simulink model "simpSubPlatform_th"  (R2018b)
settings: Solver=VariableStepAuto  StartTime=0.0  StopTime=sim_time  RelTol=1e-3
values from neighbouring files (symbols this model uses):
  Cd = 0.5    [simpSubPlatform_ts.m]
  dia_t = 0.05    [simpSubPlatform_ts.m]
  E = 3.8e9    (= 3800000000)    [simpSubPlatform_ts.m]
  flow = [.1 0 0]    [simpSubPlatform_ts.m]
  grav = 9.81    [simpSubPlatform_ts.m]
  initEulerAngles = [0 0 0]    [simpSubPlatform_ts.m]
  initPos = [0 0 100]    [simpSubPlatform_ts.m]
  mass = rho*vol/buoyF    (= 2692.30769231)    [simpSubPlatform_ts.m]
  rho = 1000    [simpSubPlatform_ts.m]
  rho_tether = 300    [simpSubPlatform_ts.m]
  tetherLengths = (norm(initPos+thr1Pt-thr1GndPos))*ones(3,1)    [simpSubPlatform_ts.m]
  thr1Pt = [0 1 -.5]    [simpSubPlatform_ts.m]
  thr2Pt = [cosd(30),-sind(30),-.5]    [simpSubPlatform_ts.m]
  thr3Pt = [-cosd(30),-sind(30),-.5]    [simpSubPlatform_ts.m]
  zeta = 0.05    [simpSubPlatform_ts.m]
undefined symbols (not defined in the file or in its folder): ini_Ri_o, ini_Vi_o, initNodePoss, initNodeVels, rotation_sequence, sim_param, singleTether_cl, Subsystem, Subsystem1, tetherBuoyancyAndWeight_ul, thr1Gnd, thr2Gnd, thr3Gnd, threeTethers_cl, zOcean
libraries: cylinderVolume_ul x3, tetherDragForce_ul x3, tetherInternalForces_ul x3, simpSubPlatform_cl x1, vectorNormalizer_ul x1
settings Model: Creator=Erin B  LastModifiedBy=Erin B

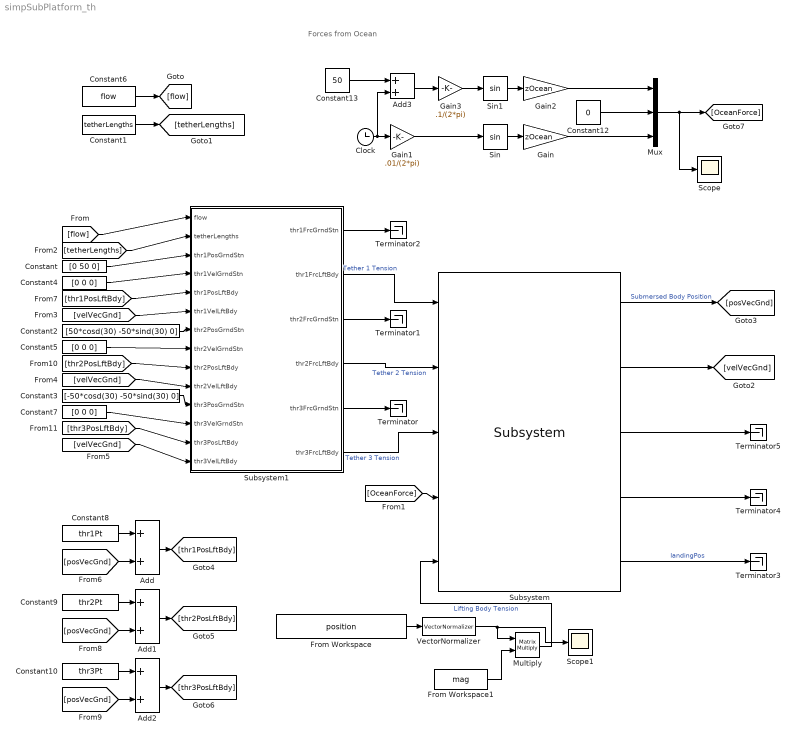
== system simpSubPlatform_th ==
  note: Forces from Ocean
  Add{,1..3} (4 alike) : Sum
  Clock : Clock
  Constant : Constant  Value=[0 50 0]
  Constant1 : Constant  Value=tetherLengths
  Constant10 : Constant  Value=thr3Pt
  Constant12 : Constant  Value=0
  Constant13 : Constant  Value=50
  Constant2 : Constant  Value=[50*cosd(30) -50*sind(30) 0]
  Constant3 : Constant  Value=[-50*cosd(30) -50*sind(30) 0]
  Constant4 : Constant  Value=[0 0 0]
  Constant5 : Constant  Value=[0 0 0]
  Constant6 : Constant  Value=flow
  Constant7 : Constant  Value=[0 0 0]
  Constant8 : Constant  Value=thr1Pt
  Constant9 : Constant  Value=thr2Pt
  From Workspace : FromWorkspace  VariableName=position  SampleTime=0
  From Workspace1 : FromWorkspace  VariableName=mag  SampleTime=0
  Gain : Gain  Gain=zOcean
  Gain1 : Gain  Gain=.01/(2*pi)
  Gain2 : Gain  Gain=zOcean
  Gain3 : Gain  Gain=.1/(2*pi)
  Multiply : Product  Multiplication=Matrix(*)
  Mux : Mux  Inputs=3
  Scope : Scope
  Scope1 : Scope
  Sin : Trigonometry  OutputSignalType=real
  Sin1 : Trigonometry  OutputSignalType=real
  Subsystem : simpSubPlatform_cl/Subsystem  SystemSampleTime=-1
  Subsystem1 : Subsystem  AncestorBlock=threeTethers_cl/Subsystem1
  Terminator{,1..5} (6 alike) : Terminator
  "VectorNormalizer " : vectorNormalizer_ul/VectorNormalizer   SystemSampleTime=-1
  wires:
  Subsystem1/4(thr2FrcLftBdy) -> Subsystem/2  "Tether 2 Tension"
  Subsystem1/5(thr3FrcGrndStn) -> Terminator/1
  Subsystem1/3(thr2FrcGrndStn) -> Terminator1/1
  Subsystem1/1(thr1FrcGrndStn) -> Terminator2/1
  Constant6/1 -> [flow]
  [flow] -> Subsystem1/1(flow)
  Constant1/1 -> [tetherLengths]
  [tetherLengths] -> Subsystem1/2(tetherLengths)
  Constant/1 -> Subsystem1/3(thr1PosGrndStn)
  Constant2/1 -> Subsystem1/7(thr2PosGrndStn)
  Constant3/1 -> Subsystem1/11(thr3PosGrndStn)
  Constant4/1 -> Subsystem1/4(thr1VelGrndStn)
  Constant5/1 -> Subsystem1/8(thr2VelGrndStn)
  Constant7/1 -> Subsystem1/12(thr3VelGrndStn)
  Subsystem/5 -> Terminator3/1  "landingPos"
  Subsystem/2 -> [velVecGnd]
  [velVecGnd] -> Subsystem1/6(thr1VelLftBdy)
  [velVecGnd] -> Subsystem1/10(thr2VelLftBdy)
  [velVecGnd] -> Subsystem1/14(thr3VelLftBdy)
  Constant8/1 -> Add/1
  Subsystem/1 -> [posVecGnd]  "Submersed Body Position"
  [posVecGnd] -> Add/2
  Add/1 -> [thr1PosLftBdy]
  [thr1PosLftBdy] -> Subsystem1/5(thr1PosLftBdy)
  Add1/1 -> [thr2PosLftBdy]
  Constant9/1 -> Add1/1
  [posVecGnd] -> Add1/2
  Add2/1 -> [thr3PosLftBdy]
  Constant10/1 -> Add2/1
  [posVecGnd] -> Add2/2
  [thr2PosLftBdy] -> Subsystem1/9(thr2PosLftBdy)
  [thr3PosLftBdy] -> Subsystem1/13(thr3PosLftBdy)
  Subsystem/4 -> Terminator4/1
  Subsystem/3 -> Terminator5/1
  Subsystem1/6(thr3FrcLftBdy) -> Subsystem/3  "Tether 3 Tension"
  Subsystem1/2(thr1FrcLftBdy) -> Subsystem/1  "Tether 1 Tension"
  Mux/1 -> Scope/1, [OceanForce]
  Sin/1 -> Gain/1
  Clock/1 -> Add3/2, Gain1/1
  [OceanForce] -> Subsystem/4
  Gain1/1 -> Sin/1
  Gain/1 -> Mux/3
  Constant13/1 -> Add3/1
  Add3/1 -> Gain3/1
  Sin1/1 -> Gain2/1
  Constant12/1 -> Mux/2
  Gain3/1 -> Sin1/1
  Gain2/1 -> Mux/1
  From Workspace/1 -> "VectorNormalizer "/1
  "VectorNormalizer "/1 -> Scope1/1, Multiply/1
  From Workspace1/1 -> Multiply/2
  Multiply/1 -> Subsystem/5  "Lifting Body Tension"

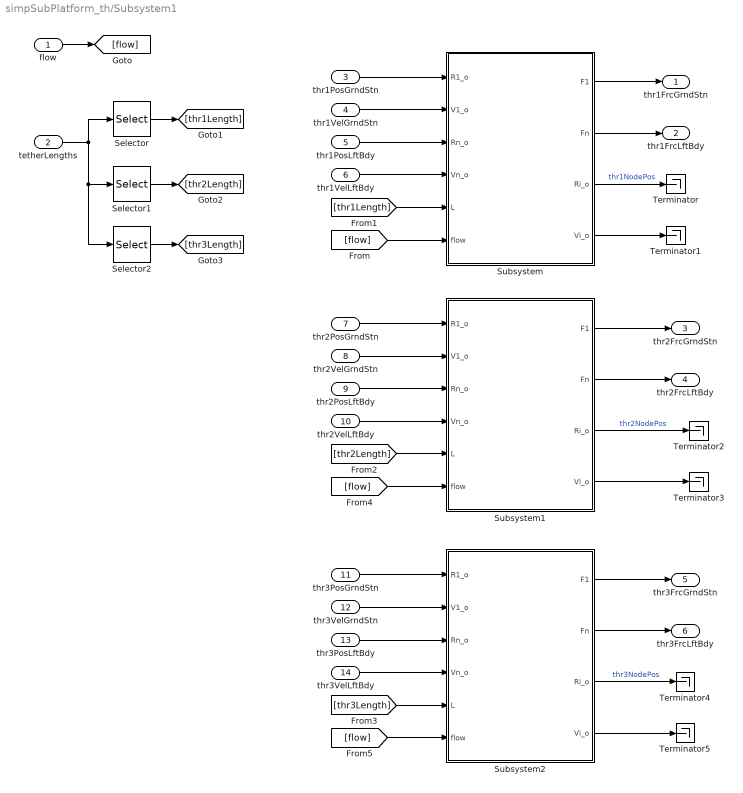
== system simpSubPlatform_th/Subsystem1 ==
  flow : Inport
  tetherLengths : Inport  Port=2
  thr1PosGrndStn : Inport  Port=3
  thr1VelGrndStn : Inport  Port=4
  thr1PosLftBdy : Inport  Port=5
  thr1VelLftBdy : Inport  Port=6
  thr2PosGrndStn : Inport  Port=7
  thr2VelGrndStn : Inport  Port=8
  thr2PosLftBdy : Inport  Port=9
  thr2VelLftBdy : Inport  Port=10
  thr3PosGrndStn : Inport  Port=11
  thr3VelGrndStn : Inport  Port=12
  thr3PosLftBdy : Inport  Port=13
  thr3VelLftBdy : Inport  Port=14
  Selector : Selector  InputPortWidth=3  IndexOptions=Index vector (dialog)  Indices=1  OutputSizes=1
  Selector1 : Selector  InputPortWidth=3  IndexOptions=Index vector (dialog)  Indices=2  OutputSizes=1
  Selector2 : Selector  InputPortWidth=3  IndexOptions=Index vector (dialog)  Indices=3  OutputSizes=1
  Subsystem : Subsystem  AncestorBlock=singleTether_cl/Subsystem  mask{N=sim_param.N, dia_t=dia_t, E=E, rho_tether=rho_tether + rho, Cd=Cd, zeta=zeta, rho=rho, g=grav, mass=mass, ini_Rn_o=initPos + (rotation_sequence(initEulerAngles)*thr1Pt')', ini_R1_o=thr1Gnd}
      mask prompts: N "Number of nodes (N>=2)"; dia_t "Tether diameter (m)"; E "Tether youngs modulus (N/m^2)"; rho_tether "Tether density (kg/m^3)"; Cd "Tether drag coefficient"; zeta "Damping ratio"; rho "Fluid density"; g "Gravitational acceleration"; mass "Vehicle mass"; ini_Rn_o "Initial vehicle attachment position vector"; ini_R1_o "Initial ground attachment position vector"
      mask init:
      | singleTether_init
      mask DialogControl Container2 Prompt: Tether properties
  Subsystem1 : Subsystem  AncestorBlock=singleTether_cl/Subsystem  mask{N=sim_param.N, dia_t=dia_t, E=E, rho_tether=rho_tether + rho, Cd=Cd, zeta=zeta, rho=rho, g=grav, mass=mass, ini_Rn_o=initPos + (rotation_sequence(initEulerAngles)*thr2Pt')', ini_R1_o=thr2Gnd}
      mask prompts: N "Number of nodes (N>=2)"; dia_t "Tether diameter (m)"; E "Tether youngs modulus (N/m^2)"; rho_tether "Tether density (kg/m^3)"; Cd "Tether drag coefficient"; zeta "Damping ratio"; rho "Fluid density"; g "Gravitational acceleration"; mass "Vehicle mass"; ini_Rn_o "Initial vehicle attachment position vector"; ini_R1_o "Initial ground attachment position vector"
      mask init:
      | singleTether_init
      mask DialogControl Container2 Prompt: Tether properties
  Subsystem2 : Subsystem  AncestorBlock=singleTether_cl/Subsystem  mask{N=sim_param.N, dia_t=dia_t, E=E, rho_tether=rho_tether + rho, Cd=Cd, zeta=zeta, rho=rho, g=grav, mass=mass, ini_Rn_o=initPos + (rotation_sequence(initEulerAngles)*thr3Pt')', ini_R1_o=thr3Gnd}
      mask prompts: N "Number of nodes (N>=2)"; dia_t "Tether diameter (m)"; E "Tether youngs modulus (N/m^2)"; rho_tether "Tether density (kg/m^3)"; Cd "Tether drag coefficient"; zeta "Damping ratio"; rho "Fluid density"; g "Gravitational acceleration"; mass "Vehicle mass"; ini_Rn_o "Initial vehicle attachment position vector"; ini_R1_o "Initial ground attachment position vector"
      mask init:
      | singleTether_init
      mask DialogControl Container2 Prompt: Tether properties
  Terminator{,1..5} (6 alike) : Terminator
  thr1FrcGrndStn : Outport
  thr1FrcLftBdy : Outport  Port=2
  thr2FrcGrndStn : Outport  Port=3
  thr2FrcLftBdy : Outport  Port=4
  thr3FrcGrndStn : Outport  Port=5
  thr3FrcLftBdy : Outport  Port=6
  wires:
  Subsystem1/1(F1) -> thr2FrcGrndStn/1
  Subsystem1/2(Fn) -> thr2FrcLftBdy/1
  Subsystem1/3(Ri_o) -> Terminator2/1  "thr2NodePos"
  Subsystem1/4(Vi_o) -> Terminator3/1
  Subsystem2/1(F1) -> thr3FrcGrndStn/1
  Subsystem2/2(Fn) -> thr3FrcLftBdy/1
  Subsystem2/3(Ri_o) -> Terminator4/1  "thr3NodePos"
  Subsystem2/4(Vi_o) -> Terminator5/1
  Subsystem/4(Vi_o) -> Terminator1/1
  Subsystem/3(Ri_o) -> Terminator/1  "thr1NodePos"
  Subsystem/2(Fn) -> thr1FrcLftBdy/1
  Subsystem/1(F1) -> thr1FrcGrndStn/1
  thr3PosGrndStn/1 -> Subsystem2/1(R1_o)
  thr3VelGrndStn/1 -> Subsystem2/2(V1_o)
  thr3PosLftBdy/1 -> Subsystem2/3(Rn_o)
  thr3VelLftBdy/1 -> Subsystem2/4(Vn_o)
  thr2VelLftBdy/1 -> Subsystem1/4(Vn_o)
  thr2PosLftBdy/1 -> Subsystem1/3(Rn_o)
  thr2VelGrndStn/1 -> Subsystem1/2(V1_o)
  thr2PosGrndStn/1 -> Subsystem1/1(R1_o)
  [flow] -> Subsystem2/6(flow)
  [flow] -> Subsystem1/6(flow)
  [thr3Length] -> Subsystem2/5(L)
  [thr2Length] -> Subsystem1/5(L)
  [thr1Length] -> Subsystem/5(L)
  Selector2/1 -> [thr3Length]
  Selector1/1 -> [thr2Length]
  tetherLengths/1 -> Selector2/1, Selector1/1, Selector/1
  Selector/1 -> [thr1Length]
  [flow] -> Subsystem/6(flow)
  flow/1 -> [flow]
  thr1PosLftBdy/1 -> Subsystem/3(Rn_o)
  thr1VelLftBdy/1 -> Subsystem/4(Vn_o)
  thr1VelGrndStn/1 -> Subsystem/2(V1_o)
  thr1PosGrndStn/1 -> Subsystem/1(R1_o)

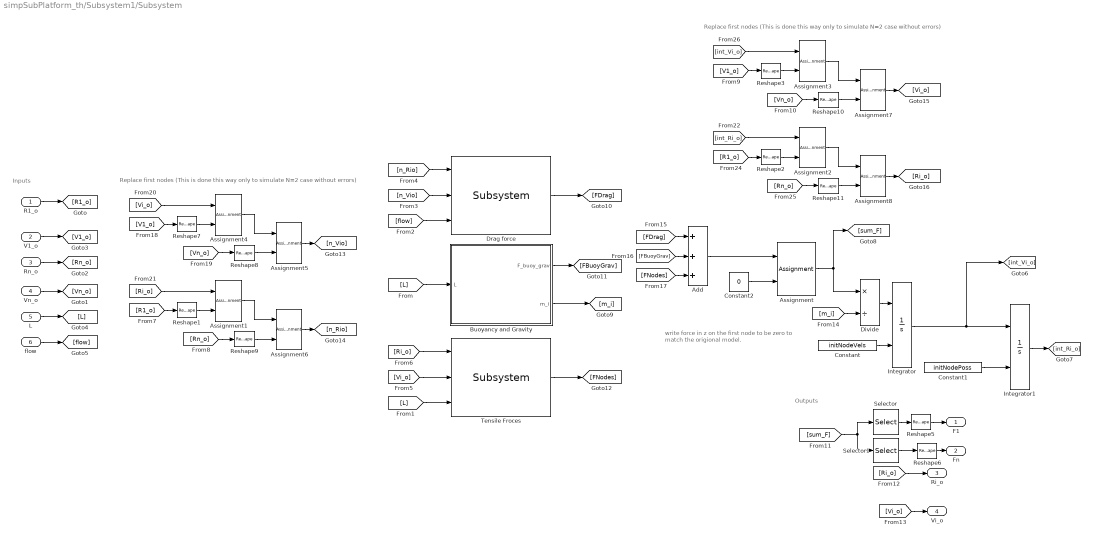
== system simpSubPlatform_th/Subsystem1/Subsystem ==
  note: write force in z on the first node to be zero
      | to match the origional model.
  note: Replace first nodes (This is done this way only to simulate N=2 case
      | without errors)
  note: Outputs
  note: Inputs
  note: Replace first nodes (This is done this way only to simulate N=2 case
      | without errors)
  R1_o : Inport
  V1_o : Inport  Port=2
  Rn_o : Inport  Port=3
  Vn_o : Inport  Port=4
  L : Inport  Port=5
  flow : Inport  Port=6
  Add : Sum  Inputs=+++
  Assignment : Assignment  NumberOfDimensions=2  DiagnosticForDimensions=Warning  IndexOptions=Index vector (dialog),Index vector (dialog)  Indices=3,1  OutputSizes=1,1
  Assignment{1..4} (4 alike) : Assignment  NumberOfDimensions=2  DiagnosticForDimensions=Warning  IndexOptions=Assign all,Index vector (dialog)  Indices=1,1  OutputSizes=1,1
  Assignment{5..8} (4 alike) : Assignment  NumberOfDimensions=2  DiagnosticForDimensions=Warning  IndexOptions=Assign all,Index vector (dialog)  Indices=1,N  OutputSizes=1,1
  Buoyancy and Gravity : Subsystem  AncestorBlock=tetherBuoyancyAndWeight_ul/Subsystem  mask{N=N, dia_t=dia_t, rho_fluid=rho, rho_tether=rho_tether, g=g}
      mask prompts: N "Number of nodes (N>=2)"; dia_t "Tether diameter (m)"; rho_fluid "Fluid density (kg/m^3)"; rho_tether "Tether density (kg/m^3)"; g "Gravitational acceleration (m/s^2)"
  Constant : Constant  Value=initNodeVels
  Constant1 : Constant  Value=initNodePoss
  Constant2 : Constant  Value=0
  Divide : Product  Inputs=*/
  Drag force : tetherDragForce_ul/Subsystem  Cd=Cd  rho_fluid=rho  dia_t=dia_t
  Integrator : Integrator  InitialConditionSource=external  InitialCondition=ini_Vi_o
  Integrator1 : Integrator  InitialConditionSource=external  InitialCondition=ini_Ri_o
  Reshape{1..3,5..11} (10 alike) : Reshape  OutputDimensionality=Column vector (2-D)
  Selector : Selector  NumberOfDimensions=2  InputPortWidth=3  IndexOptions=Select all,Index vector (dialog)  Indices=[1],1  OutputSizes=1,1
  Selector1 : Selector  NumberOfDimensions=2  InputPortWidth=3  IndexOptions=Select all,Index vector (dialog)  Indices=[N],N  OutputSizes=1,1
  Tensile Froces : tetherInternalForces_ul/Subsystem  N=N  E=E  dia_t=dia_t  mass=mass  zeta=zeta
  F1 : Outport
  Fn : Outport  Port=2
  Ri_o : Outport  Port=3
  Vi_o : Outport  Port=4
  wires:
  R1_o/1 -> [R1_o]
  V1_o/1 -> [V1_o]
  Rn_o/1 -> [Rn_o]
  Vn_o/1 -> [Vn_o]
  L/1 -> [L]
  flow/1 -> [flow]
  [L] -> Buoyancy and Gravity/1(L)
  [L] -> Tensile Froces/3
  [flow] -> Drag force/3
  Buoyancy and Gravity/1(F_buoy_grav) -> [FBuoyGrav]
  Drag force/1 -> [FDrag]
  Tensile Froces/1 -> [FNodes]
  Divide/1 -> Integrator/1
  [n_Rio] -> Drag force/1
  [Vi_o] -> Tensile Froces/2
  [Ri_o] -> Tensile Froces/1
  Integrator/1 -> [int_Vi_o], Integrator1/1
  [sum_F] -> Selector/1, Selector1/1
  [Ri_o] -> Ri_o/1
  [Vi_o] -> Vi_o/1
  Selector1/1 -> Reshape6/1
  Reshape6/1 -> Fn/1
  Selector/1 -> Reshape5/1
  Reshape5/1 -> F1/1
  Constant/1 -> Integrator/2
  Constant1/1 -> Integrator1/2
  Buoyancy and Gravity/2(m_i) -> [m_i]
  [m_i] -> Divide/2
  [FBuoyGrav] -> Add/2
  [FDrag] -> Add/1
  [FNodes] -> Add/3
  Reshape7/1 -> Assignment4/2
  [V1_o] -> Reshape7/1
  [Vi_o] -> Assignment4/1
  [Vn_o] -> Reshape8/1
  Reshape8/1 -> Assignment5/2
  Assignment4/1 -> Assignment5/1
  Assignment5/1 -> [n_Vio]
  [n_Vio] -> Drag force/2
  Assignment1/1 -> Assignment6/1
  [R1_o] -> Reshape1/1
  [Rn_o] -> Reshape9/1
  Assignment6/1 -> [n_Rio]
  [Ri_o] -> Assignment1/1
  Reshape1/1 -> Assignment1/2
  Reshape9/1 -> Assignment6/2
  Integrator1/1 -> [int_Ri_o]
  [V1_o] -> Reshape3/1
  Reshape3/1 -> Assignment3/2
  Assignment3/1 -> Assignment7/1
  Reshape11/1 -> Assignment8/2
  [int_Vi_o] -> Assignment3/1
  [R1_o] -> Reshape2/1
  [Vn_o] -> Reshape10/1
  [Rn_o] -> Reshape11/1
  Assignment7/1 -> [Vi_o]
  Assignment2/1 -> Assignment8/1
  [int_Ri_o] -> Assignment2/1
  Reshape10/1 -> Assignment7/2
  Assignment8/1 -> [Ri_o]
  Reshape2/1 -> Assignment2/2
  Assignment/1 -> [sum_F], Divide/1
  Add/1 -> Assignment/1
  Constant2/1 -> Assignment/2

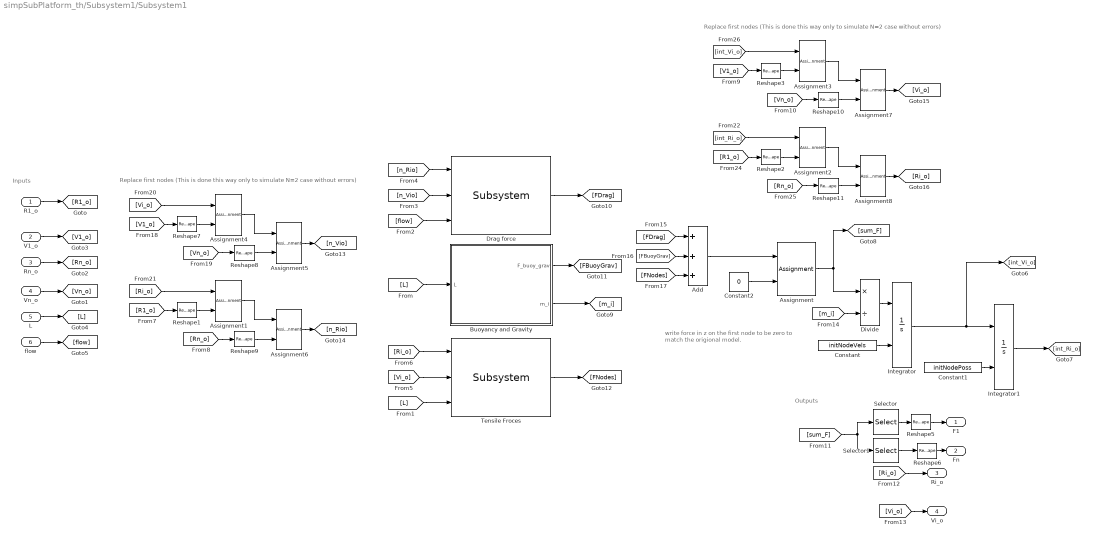
== system simpSubPlatform_th/Subsystem1/Subsystem1 ==
  note: write force in z on the first node to be zero
      | to match the origional model.
  note: Replace first nodes (This is done this way only to simulate N=2 case
      | without errors)
  note: Outputs
  note: Inputs
  note: Replace first nodes (This is done this way only to simulate N=2 case
      | without errors)
  R1_o : Inport
  V1_o : Inport  Port=2
  Rn_o : Inport  Port=3
  Vn_o : Inport  Port=4
  L : Inport  Port=5
  flow : Inport  Port=6
  Add : Sum  Inputs=+++
  Assignment : Assignment  NumberOfDimensions=2  DiagnosticForDimensions=Warning  IndexOptions=Index vector (dialog),Index vector (dialog)  Indices=3,1  OutputSizes=1,1
  Assignment{1..4} (4 alike) : Assignment  NumberOfDimensions=2  DiagnosticForDimensions=Warning  IndexOptions=Assign all,Index vector (dialog)  Indices=1,1  OutputSizes=1,1
  Assignment{5..8} (4 alike) : Assignment  NumberOfDimensions=2  DiagnosticForDimensions=Warning  IndexOptions=Assign all,Index vector (dialog)  Indices=1,N  OutputSizes=1,1
  Buoyancy and Gravity : Subsystem  AncestorBlock=tetherBuoyancyAndWeight_ul/Subsystem  mask{N=N, dia_t=dia_t, rho_fluid=rho, rho_tether=rho_tether, g=g}
      mask prompts: N "Number of nodes (N>=2)"; dia_t "Tether diameter (m)"; rho_fluid "Fluid density (kg/m^3)"; rho_tether "Tether density (kg/m^3)"; g "Gravitational acceleration (m/s^2)"
  Constant : Constant  Value=initNodeVels
  Constant1 : Constant  Value=initNodePoss
  Constant2 : Constant  Value=0
  Divide : Product  Inputs=*/
  Drag force : tetherDragForce_ul/Subsystem  Cd=Cd  rho_fluid=rho  dia_t=dia_t
  Integrator : Integrator  InitialConditionSource=external  InitialCondition=ini_Vi_o
  Integrator1 : Integrator  InitialConditionSource=external  InitialCondition=ini_Ri_o
  Reshape{1..3,5..11} (10 alike) : Reshape  OutputDimensionality=Column vector (2-D)
  Selector : Selector  NumberOfDimensions=2  InputPortWidth=3  IndexOptions=Select all,Index vector (dialog)  Indices=[1],1  OutputSizes=1,1
  Selector1 : Selector  NumberOfDimensions=2  InputPortWidth=3  IndexOptions=Select all,Index vector (dialog)  Indices=[N],N  OutputSizes=1,1
  Tensile Froces : tetherInternalForces_ul/Subsystem  N=N  E=E  dia_t=dia_t  mass=mass  zeta=zeta
  F1 : Outport
  Fn : Outport  Port=2
  Ri_o : Outport  Port=3
  Vi_o : Outport  Port=4
  wires:
  R1_o/1 -> [R1_o]
  V1_o/1 -> [V1_o]
  Rn_o/1 -> [Rn_o]
  Vn_o/1 -> [Vn_o]
  L/1 -> [L]
  flow/1 -> [flow]
  [L] -> Buoyancy and Gravity/1(L)
  [L] -> Tensile Froces/3
  [flow] -> Drag force/3
  Buoyancy and Gravity/1(F_buoy_grav) -> [FBuoyGrav]
  Drag force/1 -> [FDrag]
  Tensile Froces/1 -> [FNodes]
  Divide/1 -> Integrator/1
  [n_Rio] -> Drag force/1
  [Vi_o] -> Tensile Froces/2
  [Ri_o] -> Tensile Froces/1
  Integrator/1 -> [int_Vi_o], Integrator1/1
  [sum_F] -> Selector/1, Selector1/1
  [Ri_o] -> Ri_o/1
  [Vi_o] -> Vi_o/1
  Selector1/1 -> Reshape6/1
  Reshape6/1 -> Fn/1
  Selector/1 -> Reshape5/1
  Reshape5/1 -> F1/1
  Constant/1 -> Integrator/2
  Constant1/1 -> Integrator1/2
  Buoyancy and Gravity/2(m_i) -> [m_i]
  [m_i] -> Divide/2
  [FBuoyGrav] -> Add/2
  [FDrag] -> Add/1
  [FNodes] -> Add/3
  Reshape7/1 -> Assignment4/2
  [V1_o] -> Reshape7/1
  [Vi_o] -> Assignment4/1
  [Vn_o] -> Reshape8/1
  Reshape8/1 -> Assignment5/2
  Assignment4/1 -> Assignment5/1
  Assignment5/1 -> [n_Vio]
  [n_Vio] -> Drag force/2
  Assignment1/1 -> Assignment6/1
  [R1_o] -> Reshape1/1
  [Rn_o] -> Reshape9/1
  Assignment6/1 -> [n_Rio]
  [Ri_o] -> Assignment1/1
  Reshape1/1 -> Assignment1/2
  Reshape9/1 -> Assignment6/2
  Integrator1/1 -> [int_Ri_o]
  [V1_o] -> Reshape3/1
  Reshape3/1 -> Assignment3/2
  Assignment3/1 -> Assignment7/1
  Reshape11/1 -> Assignment8/2
  [int_Vi_o] -> Assignment3/1
  [R1_o] -> Reshape2/1
  [Vn_o] -> Reshape10/1
  [Rn_o] -> Reshape11/1
  Assignment7/1 -> [Vi_o]
  Assignment2/1 -> Assignment8/1
  [int_Ri_o] -> Assignment2/1
  Reshape10/1 -> Assignment7/2
  Assignment8/1 -> [Ri_o]
  Reshape2/1 -> Assignment2/2
  Assignment/1 -> [sum_F], Divide/1
  Add/1 -> Assignment/1
  Constant2/1 -> Assignment/2

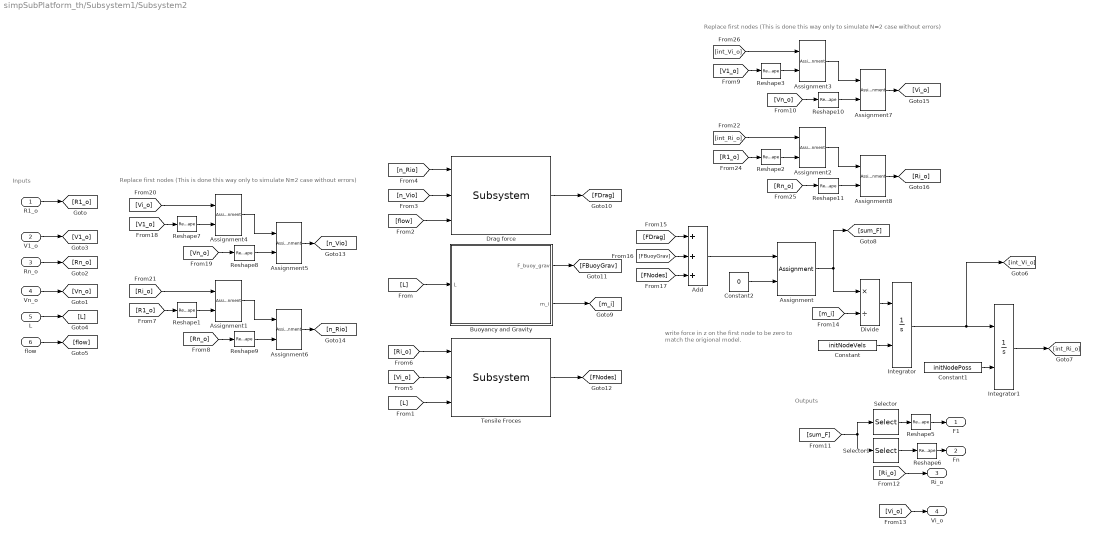
== system simpSubPlatform_th/Subsystem1/Subsystem2 ==
  note: write force in z on the first node to be zero
      | to match the origional model.
  note: Replace first nodes (This is done this way only to simulate N=2 case
      | without errors)
  note: Outputs
  note: Inputs
  note: Replace first nodes (This is done this way only to simulate N=2 case
      | without errors)
  R1_o : Inport
  V1_o : Inport  Port=2
  Rn_o : Inport  Port=3
  Vn_o : Inport  Port=4
  L : Inport  Port=5
  flow : Inport  Port=6
  Add : Sum  Inputs=+++
  Assignment : Assignment  NumberOfDimensions=2  DiagnosticForDimensions=Warning  IndexOptions=Index vector (dialog),Index vector (dialog)  Indices=3,1  OutputSizes=1,1
  Assignment{1..4} (4 alike) : Assignment  NumberOfDimensions=2  DiagnosticForDimensions=Warning  IndexOptions=Assign all,Index vector (dialog)  Indices=1,1  OutputSizes=1,1
  Assignment{5..8} (4 alike) : Assignment  NumberOfDimensions=2  DiagnosticForDimensions=Warning  IndexOptions=Assign all,Index vector (dialog)  Indices=1,N  OutputSizes=1,1
  Buoyancy and Gravity : Subsystem  AncestorBlock=tetherBuoyancyAndWeight_ul/Subsystem  mask{N=N, dia_t=dia_t, rho_fluid=rho, rho_tether=rho_tether, g=g}
      mask prompts: N "Number of nodes (N>=2)"; dia_t "Tether diameter (m)"; rho_fluid "Fluid density (kg/m^3)"; rho_tether "Tether density (kg/m^3)"; g "Gravitational acceleration (m/s^2)"
  Constant : Constant  Value=initNodeVels
  Constant1 : Constant  Value=initNodePoss
  Constant2 : Constant  Value=0
  Divide : Product  Inputs=*/
  Drag force : tetherDragForce_ul/Subsystem  Cd=Cd  rho_fluid=rho  dia_t=dia_t
  Integrator : Integrator  InitialConditionSource=external  InitialCondition=ini_Vi_o
  Integrator1 : Integrator  InitialConditionSource=external  InitialCondition=ini_Ri_o
  Reshape{1..3,5..11} (10 alike) : Reshape  OutputDimensionality=Column vector (2-D)
  Selector : Selector  NumberOfDimensions=2  InputPortWidth=3  IndexOptions=Select all,Index vector (dialog)  Indices=[1],1  OutputSizes=1,1
  Selector1 : Selector  NumberOfDimensions=2  InputPortWidth=3  IndexOptions=Select all,Index vector (dialog)  Indices=[N],N  OutputSizes=1,1
  Tensile Froces : tetherInternalForces_ul/Subsystem  N=N  E=E  dia_t=dia_t  mass=mass  zeta=zeta
  F1 : Outport
  Fn : Outport  Port=2
  Ri_o : Outport  Port=3
  Vi_o : Outport  Port=4
  wires:
  R1_o/1 -> [R1_o]
  V1_o/1 -> [V1_o]
  Rn_o/1 -> [Rn_o]
  Vn_o/1 -> [Vn_o]
  L/1 -> [L]
  flow/1 -> [flow]
  [L] -> Buoyancy and Gravity/1(L)
  [L] -> Tensile Froces/3
  [flow] -> Drag force/3
  Buoyancy and Gravity/1(F_buoy_grav) -> [FBuoyGrav]
  Drag force/1 -> [FDrag]
  Tensile Froces/1 -> [FNodes]
  Divide/1 -> Integrator/1
  [n_Rio] -> Drag force/1
  [Vi_o] -> Tensile Froces/2
  [Ri_o] -> Tensile Froces/1
  Integrator/1 -> [int_Vi_o], Integrator1/1
  [sum_F] -> Selector/1, Selector1/1
  [Ri_o] -> Ri_o/1
  [Vi_o] -> Vi_o/1
  Selector1/1 -> Reshape6/1
  Reshape6/1 -> Fn/1
  Selector/1 -> Reshape5/1
  Reshape5/1 -> F1/1
  Constant/1 -> Integrator/2
  Constant1/1 -> Integrator1/2
  Buoyancy and Gravity/2(m_i) -> [m_i]
  [m_i] -> Divide/2
  [FBuoyGrav] -> Add/2
  [FDrag] -> Add/1
  [FNodes] -> Add/3
  Reshape7/1 -> Assignment4/2
  [V1_o] -> Reshape7/1
  [Vi_o] -> Assignment4/1
  [Vn_o] -> Reshape8/1
  Reshape8/1 -> Assignment5/2
  Assignment4/1 -> Assignment5/1
  Assignment5/1 -> [n_Vio]
  [n_Vio] -> Drag force/2
  Assignment1/1 -> Assignment6/1
  [R1_o] -> Reshape1/1
  [Rn_o] -> Reshape9/1
  Assignment6/1 -> [n_Rio]
  [Ri_o] -> Assignment1/1
  Reshape1/1 -> Assignment1/2
  Reshape9/1 -> Assignment6/2
  Integrator1/1 -> [int_Ri_o]
  [V1_o] -> Reshape3/1
  Reshape3/1 -> Assignment3/2
  Assignment3/1 -> Assignment7/1
  Reshape11/1 -> Assignment8/2
  [int_Vi_o] -> Assignment3/1
  [R1_o] -> Reshape2/1
  [Vn_o] -> Reshape10/1
  [Rn_o] -> Reshape11/1
  Assignment7/1 -> [Vi_o]
  Assignment2/1 -> Assignment8/1
  [int_Ri_o] -> Assignment2/1
  Reshape10/1 -> Assignment7/2
  Assignment8/1 -> [Ri_o]
  Reshape2/1 -> Assignment2/2
  Assignment/1 -> [sum_F], Divide/1
  Add/1 -> Assignment/1
  Constant2/1 -> Assignment/2

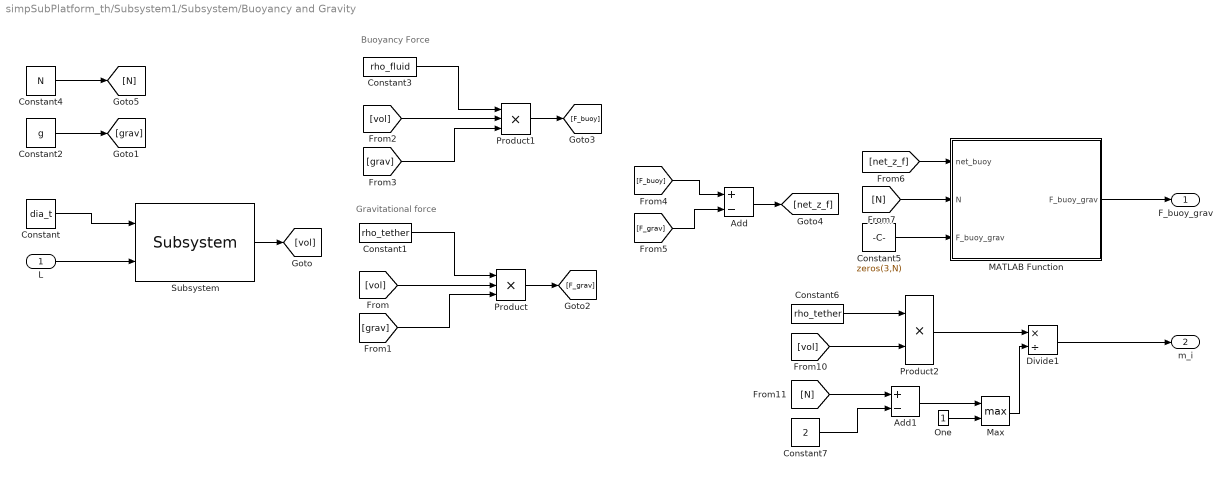
== system simpSubPlatform_th/Subsystem1/Subsystem/Buoyancy and Gravity ==
  note: Gravitational force
  note: Buoyancy Force
  L : Inport
  Add : Sum  Inputs=+-
  Add1 : Sum  Inputs=+-
  Constant : Constant  Value=dia_t
  Constant1 : Constant  Value=rho_tether
  Constant2 : Constant  Value=g
  Constant3 : Constant  Value=rho_fluid
  Constant4 : Constant  Value=N
  Constant5 : Constant  Value=zeros(3,N)
  Constant6 : Constant  Value=rho_tether
  Constant7 : Constant  Value=2
  Divide1 : Product  Inputs=*/
  MATLAB Function : MATLAB Function  TreatAsAtomicUnit=on
  Max : MinMax  Function=max  Inputs=2
  One : Constant  OutDataTypeStr=Inherit: Inherit via back propagation
  Product : Product  Inputs=3
  Product1 : Product  Inputs=3
  Product2 : Product
  Subsystem : cylinderVolume_ul/Subsystem  SystemSampleTime=-1
  F_buoy_grav : Outport
  m_i : Outport  Port=2
  wires:
  Constant7/1 -> Add1/2
  [N] -> Add1/1
  Divide1/1 -> m_i/1
  Product2/1 -> Divide1/1
  Constant6/1 -> Product2/1
  [vol] -> Product2/2
  MATLAB Function/1(F_buoy_grav) -> F_buoy_grav/1
  Constant5/1 -> MATLAB Function/3("F_buoy_grav ")
  [N] -> MATLAB Function/2(N)
  Constant4/1 -> [N]
  [net_z_f] -> MATLAB Function/1(net_buoy)
  Add/1 -> [net_z_f]
  [F_grav] -> Add/2
  [F_buoy] -> Add/1
  Product1/1 -> [F_buoy]
  [vol] -> Product1/2
  Constant3/1 -> Product1/1
  [grav] -> Product1/3
  Product/1 -> [F_grav]
  [grav] -> Product/3
  [vol] -> Product/2
  Constant1/1 -> Product/1
  Constant2/1 -> [grav]
  Subsystem/1 -> [vol]
  Constant/1 -> Subsystem/1
  L/1 -> Subsystem/2
  Max/1 -> Divide1/2
  Add1/1 -> Max/1
  One/1 -> Max/2

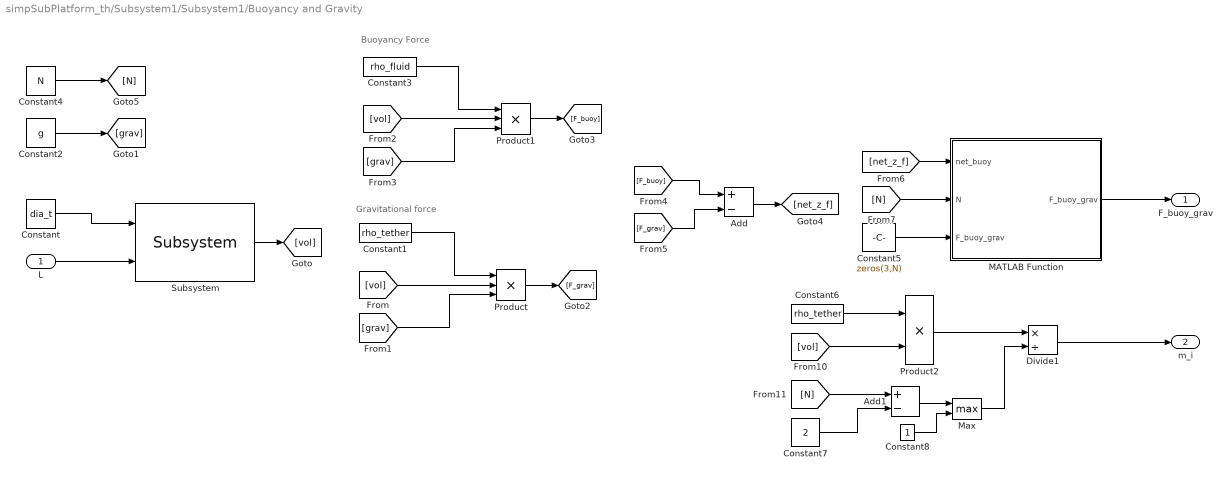
== system simpSubPlatform_th/Subsystem1/Subsystem1/Buoyancy and Gravity ==
  note: Gravitational force
  note: Buoyancy Force
  L : Inport
  Add : Sum  Inputs=+-
  Add1 : Sum  Inputs=+-
  Constant : Constant  Value=dia_t
  Constant1 : Constant  Value=rho_tether
  Constant2 : Constant  Value=g
  Constant3 : Constant  Value=rho_fluid
  Constant4 : Constant  Value=N
  Constant5 : Constant  Value=zeros(3,N)
  Constant6 : Constant  Value=rho_tether
  Constant7 : Constant  Value=2
  Constant8 : Constant
  Divide1 : Product  Inputs=*/
  MATLAB Function : MATLAB Function  TreatAsAtomicUnit=on
  Max : MinMax  Function=max  Inputs=2
  Product : Product  Inputs=3
  Product1 : Product  Inputs=3
  Product2 : Product
  Subsystem : cylinderVolume_ul/Subsystem  SystemSampleTime=-1
  F_buoy_grav : Outport
  m_i : Outport  Port=2
  wires:
  Constant7/1 -> Add1/2
  Add1/1 -> Max/1
  [N] -> Add1/1
  Divide1/1 -> m_i/1
  Product2/1 -> Divide1/1
  Constant6/1 -> Product2/1
  [vol] -> Product2/2
  MATLAB Function/1(F_buoy_grav) -> F_buoy_grav/1
  Constant5/1 -> MATLAB Function/3("F_buoy_grav ")
  [N] -> MATLAB Function/2(N)
  Constant4/1 -> [N]
  [net_z_f] -> MATLAB Function/1(net_buoy)
  Add/1 -> [net_z_f]
  [F_grav] -> Add/2
  [F_buoy] -> Add/1
  Product1/1 -> [F_buoy]
  [vol] -> Product1/2
  Constant3/1 -> Product1/1
  [grav] -> Product1/3
  Product/1 -> [F_grav]
  [grav] -> Product/3
  [vol] -> Product/2
  Constant1/1 -> Product/1
  Constant2/1 -> [grav]
  Subsystem/1 -> [vol]
  Constant/1 -> Subsystem/1
  L/1 -> Subsystem/2
  Constant8/1 -> Max/2
  Max/1 -> Divide1/2

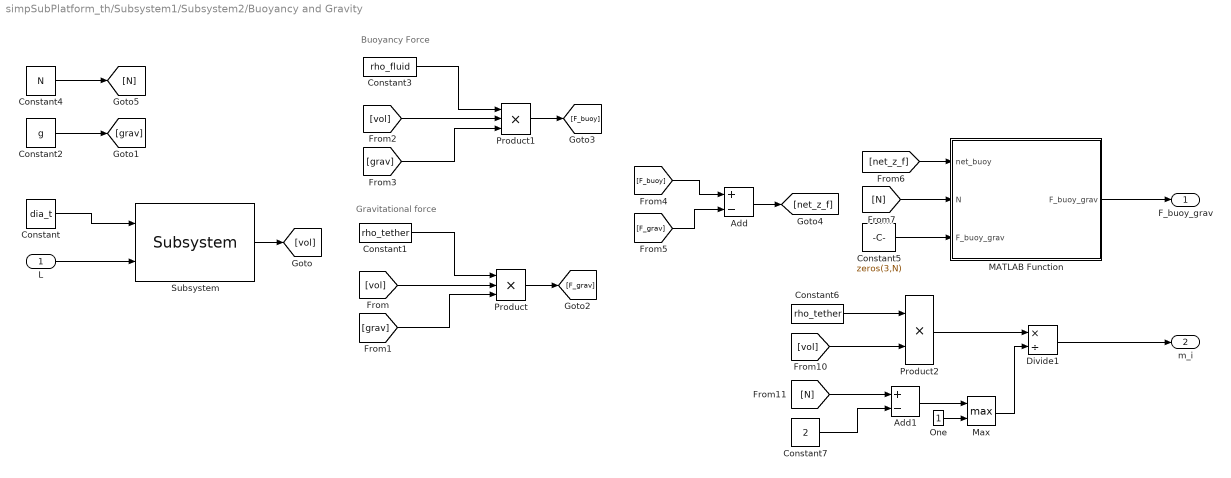
== system simpSubPlatform_th/Subsystem1/Subsystem2/Buoyancy and Gravity ==
  note: Gravitational force
  note: Buoyancy Force
  L : Inport
  Add : Sum  Inputs=+-
  Add1 : Sum  Inputs=+-
  Constant : Constant  Value=dia_t
  Constant1 : Constant  Value=rho_tether
  Constant2 : Constant  Value=g
  Constant3 : Constant  Value=rho_fluid
  Constant4 : Constant  Value=N
  Constant5 : Constant  Value=zeros(3,N)
  Constant6 : Constant  Value=rho_tether
  Constant7 : Constant  Value=2
  Divide1 : Product  Inputs=*/
  MATLAB Function : MATLAB Function  TreatAsAtomicUnit=on
  Max : MinMax  Function=max  Inputs=2
  One : Constant  OutDataTypeStr=Inherit: Inherit via back propagation
  Product : Product  Inputs=3
  Product1 : Product  Inputs=3
  Product2 : Product
  Subsystem : cylinderVolume_ul/Subsystem  SystemSampleTime=-1
  F_buoy_grav : Outport
  m_i : Outport  Port=2
  wires:
  Constant7/1 -> Add1/2
  [N] -> Add1/1
  Divide1/1 -> m_i/1
  Product2/1 -> Divide1/1
  Constant6/1 -> Product2/1
  [vol] -> Product2/2
  MATLAB Function/1(F_buoy_grav) -> F_buoy_grav/1
  Constant5/1 -> MATLAB Function/3("F_buoy_grav ")
  [N] -> MATLAB Function/2(N)
  Constant4/1 -> [N]
  [net_z_f] -> MATLAB Function/1(net_buoy)
  Add/1 -> [net_z_f]
  [F_grav] -> Add/2
  [F_buoy] -> Add/1
  Product1/1 -> [F_buoy]
  [vol] -> Product1/2
  Constant3/1 -> Product1/1
  [grav] -> Product1/3
  Product/1 -> [F_grav]
  [grav] -> Product/3
  [vol] -> Product/2
  Constant1/1 -> Product/1
  Constant2/1 -> [grav]
  Subsystem/1 -> [vol]
  Constant/1 -> Subsystem/1
  L/1 -> Subsystem/2
  Add1/1 -> Max/1
  Max/1 -> Divide1/2
  One/1 -> Max/2

== matlab function simpSubPlatform_th/Subsystem1/Subsystem1/Buoyancy and Gravity/MATLAB Function ==
  data: net_buoy input; F_buoy_grav output; N input; F_buoy_grav input
function F_buoy_grav = fcn(net_buoy,N,F_buoy_grav)

for i = 1:N
    if i == 1
        F_buoy_grav(:,i) = zeros(3,1);
    elseif i>1 && i<N
        F_buoy_grav(:,i) = net_buoy/(N-2)*[0; 0; 1];
    elseif i == N
        F_buoy_grav(:,i) = zeros(3,1);
    end
    
end

end

== matlab function simpSubPlatform_th/Subsystem1/Subsystem2/Buoyancy and Gravity/MATLAB Function ==
  data: net_buoy input; F_buoy_grav output; N input; F_buoy_grav input
function F_buoy_grav = fcn(net_buoy,N,F_buoy_grav)

for i = 1:N
    if i == 1
        F_buoy_grav(:,i) = zeros(3,1);
    elseif i>1 && i<N
        F_buoy_grav(:,i) = net_buoy/(N-2)*[0; 0; 1];
    elseif i == N
        F_buoy_grav(:,i) = zeros(3,1);
    end
    
end

end

== matlab function simpSubPlatform_th/Subsystem1/Subsystem/Buoyancy and Gravity/MATLAB Function ==
  data: net_buoy input; F_buoy_grav output; N input; F_buoy_grav input
function F_buoy_grav = fcn(net_buoy,N,F_buoy_grav)

for i = 1:N
    if i == 1
        F_buoy_grav(:,i) = zeros(3,1);
    elseif i>1 && i<N
        F_buoy_grav(:,i) = net_buoy/(N-2)*[0; 0; 1];
    elseif i == N
        F_buoy_grav(:,i) = zeros(3,1);
    end
    
end

end
